simulink model "A_Robot_2_0_m_5_V22_SI"  (R2025b)
settings: Solver=VariableStepAuto  StartTime=0.0  StopTime=150  RelTol=1e-3
model workspace (MAT data in the model file):
  Km = [1; 1]
values from neighbouring files (symbols this model uses):
  kcl = kil + 50    (= 75)    [A_init_0.m]    (also in A_init_0_v2.m; A_init_1_v2.m)
  kcr = kir + 50    (= 75)    [A_init_0.m]    (also in A_init_0_v2.m; A_init_1_v2.m)
  kil = 25    [A_init_0.m]    (also in A_init_0_v2.m; A_init_1_v2.m)
  kir = 25    [A_init_0.m]    (also in A_init_0_v2.m; A_init_1_v2.m)
  kpl = 5    [A_init_0.m]    (also in A_init_0_v2.m; A_init_1_v2.m)
  kpr = 5    [A_init_0.m]    (also in A_init_0_v2.m; A_init_1_v2.m)
  theta0 = theta_0_min + (theta_0_max - theta_0_min) * rand()    [A_init_0.m]    (also in A_init_0_v2.m; A_init_1_v2.m)
  theta_gsr = theta_gsr_min + (theta_gsr_max - theta_gsr_min) * rand()    [A_init_0.m]    (also in A_init_0_v2.m; A_init_1_v2.m)
  v_rand = v_rand_0 + (v_rand_max - v_rand_0) * rand()    [A_init_0.m]    (also in A_init_0_v2.m; A_init_1_v2.m)
  x0 = x_0_min + (x_0_max - x_0_min) * rand()    [A_init_0.m]    (also in A_init_0_v2.m; A_init_1_v2.m)
  x_gsr = x_gsr_min + (x_gsr_max - x_gsr_min) * rand()    [A_init_0.m]    (also in A_init_0_v2.m; A_init_1_v2.m)
  y0 = y_0_min + (y_0_max - y_0_min) * rand()    [A_init_0.m]    (also in A_init_0_v2.m; A_init_1_v2.m)
  y_gsr = y_gsr_min + (y_gsr_max - y_gsr_min) * rand()    [A_init_0.m]    (also in A_init_0_v2.m; A_init_1_v2.m)
undefined symbols (not defined in the file or in its folder): DiscIntNeverNeededParam
libraries: simulink x15, rllib x1
(part 1 of 3)
settings Model: PacingRate=10  Creator=rafci  LastModifiedBy=rafci
settings DataIOCC: InspectSignalLogs=on
settings DebuggingCC: AlgebraicLoopMsg=none

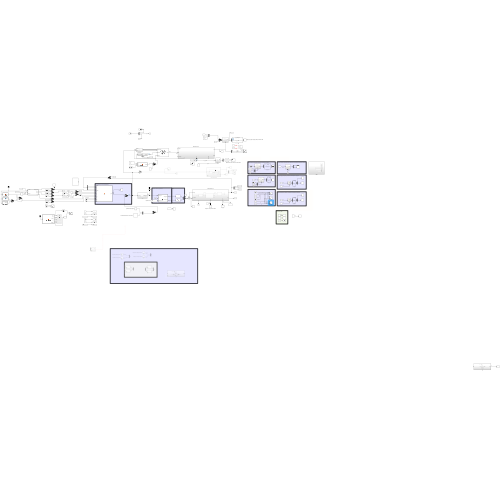
[thumbnail: Simulink's stored preview of the top-level diagram]
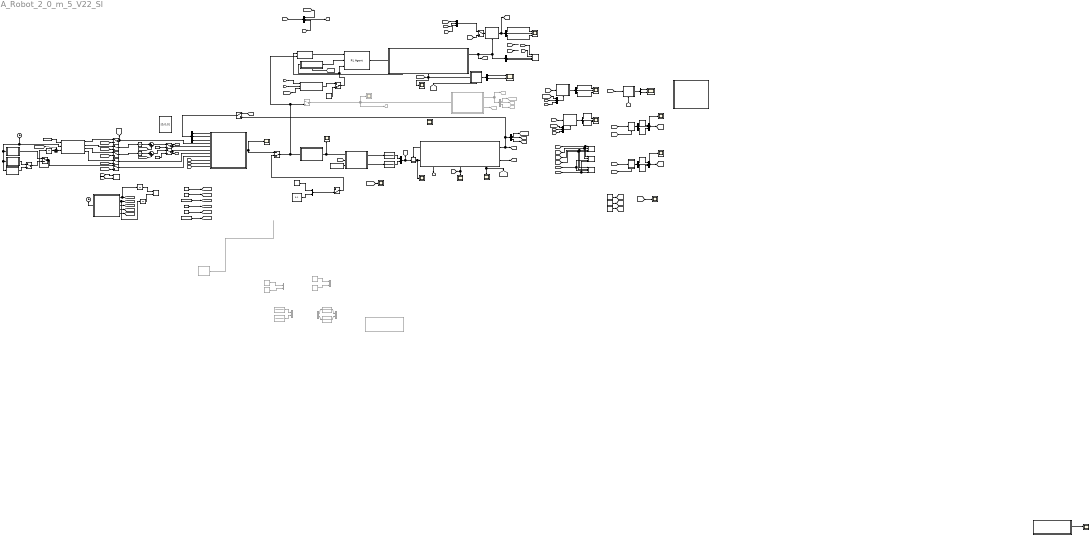
== system A_Robot_2_0_m_5_V22_SI ==
  note: Wykresy XY
  note: Błąd pozycji pomiędzy modelem kinematyki a GSR
  note: Błąd pozycji pomiędzy modelem kinematyki a pełnym
  note: Roznica napięć pomiędzy sterowaniem kinematyki a pełnego modelu
  note: $\Omega_{dsF}$
  note: FIltry
  note: parametry ASP
  note: Kinematyczny steownik platformy
  note: Blok sterowania prędkości
  note: Błąd prędkości pomiędzy modelem kinematyki a pełnym
  note: Błąd pozycji pomiędzy pełnym modelem a GSR
  Błąd napięć między pełnym modelem a NN : Scope  NumInputPorts=2
      settings: ActiveDisplayYMinimum=-28.46005  ActiveDisplayYMaximum=16.49556
  Błąd pozycji i kąta między (switch) modelem a NN : Scope  NumInputPorts=3
      settings: ActiveDisplayYMinimum=-0.50596  ActiveDisplayYMaximum=0.10747
  Clock : Clock
  Clock1 : Clock
  Constant : Constant  Value=10  VectorParams1D=off
  Constant1 : Constant  Value=40
  Constant10 : Constant  Value=x_gsr
  Constant11 : Constant  Value=y_gsr
  Constant12 : Constant  Value=theta_gsr
  Constant13 : Constant  Value=[0;0;0]
  Constant2 : Constant  Value=27
  Constant3 : Constant  Value=x0
  Constant4 : Constant  Value=y0
  Constant5 : Constant  Value=0  OutDataTypeStr=boolean
  Constant6 : Constant  Value=theta0
  Constant7 : Constant  Value=-0.5
  Constant8 : Constant  Value=-0.5
  Constant9 : Constant  Value=v_rand
  Demux : Demux  Commented=on  Outputs=3
  Demux{1..3,5,7..9,11..12} (9 alike) : Demux  Outputs=3
  Demux13 : Demux  Outputs=2
  Demux4 : Demux  Commented=on  Outputs=2
  Demux6 : Demux  Outputs=2
  Goto11 : Goto  Commented=on  GotoTag=U_k  TagVisibility=global
  Goto12 : Goto  Commented=on  GotoTag=q_k  TagVisibility=global
  Goto16 : Goto  Commented=on  GotoTag=q_d_k  TagVisibility=global
  Goto17 : Goto  Commented=on  GotoTag=theta_k  TagVisibility=global
  Goto18 : Goto  Commented=on  GotoTag=x_k  TagVisibility=global
  Goto19 : Goto  Commented=on  GotoTag=y_k  TagVisibility=global
  Integrator{,1,6..8} (5 alike) : Integrator
  J^-1 : Subsystem
  MATLAB Function : MATLAB Function  TreatAsAtomicUnit=on
  MATLAB Function1 : MATLAB Function  TreatAsAtomicUnit=on
  MATLAB Function10 : MATLAB Function  TreatAsAtomicUnit=on
  MATLAB Function2 : MATLAB Function  TreatAsAtomicUnit=on
  MATLAB Function3 : MATLAB Function  TreatAsAtomicUnit=on
  MATLAB Function6 : MATLAB Function  TreatAsAtomicUnit=on
  MATLAB Function7 : MATLAB Function  TreatAsAtomicUnit=on
  MATLAB Function9 : MATLAB Function  TreatAsAtomicUnit=on
  Manual Switch{,2..3,5..10,12,15} (11 alike) : ManualSwitch
  Manual Switch11 : ManualSwitch  CurrentSetting=0
  Manual Switch13 : ManualSwitch  Commented=on
  Manual Switch14 : ManualSwitch  CurrentSetting=0
  Manual Switch4 : ManualSwitch  CurrentSetting=0
  Model Robota 2.0 : Subsystem
      settings: PortSchema="{\"entries\":[{\"content\":{\"sides\":[{\"content\":{\"connectorIds\":[\"Out6\",\"In1\"]},\"type\":\"ConnectorPlacement.EquallySpacedRectSide\",\"uuid\":\"c09d05f6-15bd-4af9-8cdd-7798699522a1\"},{\"content\":{\"connectorIds\":[\"Out1\",\"Out2\"],\"side\":\"RIGHT\"},\"type\":\"ConnectorPlacement.EquallySpacedRectSide\",\"uuid\":\"5078d491-052a-42da-8be8-27dff9332d53\"},{\"content\":{\"side\":\"TOP\"},\"type\":\"ConnectorPlacement.EquallySpacedRectSide\",\"uuid\":\"ce1dd30c-527c-4a1c-9b39-bff6482988ba\"},{\"content\":{\"connectorIds\":[\"Out3\",\"Out4\",\"Out5\"],\"side\":\"BOTTOM\"},\"type\":\"ConnectorPlacement.EquallySpacedRectSide\",\"uuid\":\"43230f6c-2d05-4ed1-a059-067bd37565f0\"}]},\"type\":\"ConnectorPlacement.EquallySpacedConnector\",\"uuid\":\"daca06f7-ab0b-4c67-a969-f3b079c7dee2\"}],\"packageUris\":[\"http://schema.mathworks.com/mf0/Connector/R2020b\"],\"version\":\"1.0\"}"
  Model Robota 2.1 : Subsystem
      settings: PortSchema="{\"entries\":[{\"content\":{\"sides\":[{\"content\":{\"connectorIds\":[\"Out6\",\"In1\",\"In2\"]},\"type\":\"ConnectorPlacement.EquallySpacedRectSide\",\"uuid\":\"c09d05f6-15bd-4af9-8cdd-7798699522a1\"},{\"content\":{\"connectorIds\":[\"Out1\",\"Out2\"],\"side\":\"RIGHT\"},\"type\":\"ConnectorPlacement.EquallySpacedRectSide\",\"uuid\":\"5078d491-052a-42da-8be8-27dff9332d53\"},{\"content\":{\"side\":\"TOP\"},\"type\":\"ConnectorPlacement.EquallySpacedRectSide\",\"uuid\":\"ce1dd30c-527c-4a1c-9b39-bff6482988ba\"},{\"content\":{\"connectorIds\":[\"Out3\",\"Out4\",\"Out5\"],\"side\":\"BOTTOM\"},\"type\":\"ConnectorPlacement.EquallySpacedRectSide\",\"uuid\":\"43230f6c-2d05-4ed1-a059-067bd37565f0\"}]},\"type\":\"ConnectorPlacement.EquallySpacedConnector\",\"uuid\":\"daca06f7-ab0b-4c67-a969-f3b079c7dee2\"}],\"packageUris\":[\"http://schema.mathworks.com/mf0/Connector/R2020b\"],\"version\":\"1.0\"}"
  Model kinematyki1 : Subsystem  Commented=on
  Mux1 : Mux  Inputs=2
  Mux{3,6,8,10} (4 alike) : Mux  Commented=on  Inputs=2
  Mux{4..5,7,9,12} (5 alike) : Mux  Inputs=3
  Mux2 : Mux  Inputs=2
  Nagroda : Subsystem
      settings: PortSchema="{\"entries\":[{\"content\":{\"sides\":[{\"content\":{\"connectorIds\":[\"In1\"]},\"type\":\"ConnectorPlacement.EquallySpacedRectSide\",\"uuid\":\"a2f775dc-59c4-4717-86d2-15fa652a3e96\"},{\"content\":{\"connectorIds\":[\"Out1\"],\"side\":\"RIGHT\"},\"type\":\"ConnectorPlacement.EquallySpacedRectSide\",\"uuid\":\"245f7467-b166-487e-99c9-5f03cfbee592\"},{\"content\":{\"side\":\"TOP\"},\"type\":\"ConnectorPlacement.EquallySpacedRectSide\",\"uuid\":\"946a6bdb-83a2-4b9a-b4f9-a3cb3678f859\"},{\"content\":{\"connectorIds\":[\"In2\"],\"side\":\"BOTTOM\"},\"type\":\"ConnectorPlacement.EquallySpacedRectSide\",\"uuid\":\"f1f94bb1-6799-4829-990b-56c54b864c73\"}]},\"type\":\"ConnectorPlacement.EquallySpacedConnector\",\"uuid\":\"54b4897f-7a99-44dc-b2f7-11c656f05ccb\"}],\"packageUris\":[\"http://schema.mathworks.com/mf0/Connector/R2020b\"],\"version\":\"1.0\"}"
  Napięcie na lewym silniku : Constant  Commented=on  Value=12
  "Napięcie na prawym silniku " : Constant  Commented=on  Value=70
  Napięcie na wejsciowe silników : Scope
      settings: ActiveDisplayYMinimum=-5.36622  ActiveDisplayYMaximum=6.84937  DataLoggingVariableName=ScopeData8
  Obsrwacja : Subsystem
  Prędkość Lewego wału : Constant  Commented=on  Value=0
  Prędkość max : Constant  Value=161.77*2*pi
  Prędkość prawego wału : Constant  Commented=on  Value=75
  RL Agent : rllib/RL Agent  Agent=agent  ExternalActionAsInput=off  ProvideLastAction=off  ProvideCumRwd=off  TreatAsDirectFeedthrough=on  UseStrictObservationDataTypes=off
  Scope{,1..3,5..6,8,11,17,20} (10 alike) : Scope
      Scope1 settings: ActiveDisplayYMinimum=-0.01608  ActiveDisplayYMaximum=0.01608  DataLoggingVariableName=ScopeData7
      Scope11 settings: ActiveDisplayYMinimum=-0.23934  ActiveDisplayYMaximum=0.23817  DataLoggingVariableName=ScopeData7
      Scope17 settings: ActiveDisplayYMinimum=-2.83473  ActiveDisplayYMaximum=3.59922
      Scope2 settings: ActiveDisplayYMinimum=-0.01608  ActiveDisplayYMaximum=0.01608  DataLoggingVariableName=ScopeData10
      Scope20 settings: ActiveDisplayYMinimum=-0.01395  ActiveDisplayYMaximum=0.11266  DataLoggingVariableName=ScopeData2
      Scope3 settings: ActiveDisplayYMinimum=-0.0233  ActiveDisplayYMaximum=0.04203
      Scope5 settings: ActiveDisplayYMinimum=-6.16909  ActiveDisplayYMaximum=6.96286  DataLoggingVariableName=ScopeData2
      Scope6 settings: ActiveDisplayYMinimum=2.8655866160988808  ActiveDisplayYMaximum=3.93364068120718
      Scope8 settings: ActiveDisplayYMinimum=-0.02162  ActiveDisplayYMaximum=0.2946
      Scope settings: ActiveDisplayYMinimum=-0.48296536475593865  ActiveDisplayYMaximum=4.3057020124132714
  Scope12 : Scope  Commented=on
      settings: ActiveDisplayYMinimum=-0.0125  ActiveDisplayYMaximum=0.1125  DataLoggingVariableName=ScopeData8
  Scope24 : Scope  NumInputPorts=3
      settings: ActiveDisplayYMinimum=-0.06798  ActiveDisplayYMaximum=0.06446  DataLoggingVariableName=ScopeData5
  Scope4 : Scope  NumInputPorts=3
      settings: ActiveDisplayYMinimum=-0.1993  ActiveDisplayYMaximum=0.19665
  Scope9 : Scope  NumInputPorts=2
      settings: ActiveDisplayYMinimum=-0.4921  ActiveDisplayYMaximum=2.2769  DataLoggingVariableName=ScopeData6
  Stałe : Subsystem
  Subsystem : Subsystem  Commented=on
  Subsystem1 : Subsystem  Commented=on
      settings: PortSchema="{\"entries\":[{\"content\":{\"sides\":[{\"content\":{\"connectorIds\":[\"In1\"]},\"type\":\"ConnectorPlacement.EquallySpacedRectSide\",\"uuid\":\"f81facd5-8dce-4a5d-a044-cb75bd1df10e\"},{\"content\":{\"connectorIds\":[\"Out1\"],\"side\":\"RIGHT\"},\"type\":\"ConnectorPlacement.EquallySpacedRectSide\",\"uuid\":\"361c4912-9b0e-4ff4-a4c3-0f951cd83b7e\"},{\"content\":{\"side\":\"TOP\"},\"type\":\"ConnectorPlacement.EquallySpacedRectSide\",\"uuid\":\"7c64f9f2-ca51-41c2-8f6b-bbae03c31185\"},{\"content\":{\"connectorIds\":[\"In2\"],\"side\":\"BOTTOM\"},\"type\":\"ConnectorPlacement.EquallySpacedRectSide\",\"uuid\":\"00962904-9a33-4c86-93c6-1e958d83cf78\"}]},\"type\":\"ConnectorPlacement.EquallySpacedConnector\",\"uuid\":\"b3c5fd64-8318-4fc9-b064-dcb9a80ffa17\"}],\"packageUris\":[\"http://schema.mathworks.com/mf0/Connector/R2020b\"],\"version\":\"1.0\"}"
  Subsystem10 : Subsystem
      settings: PortSchema="{\"entries\":[{\"content\":{\"sides\":[{\"content\":{\"connectorIds\":[\"In1\"]},\"type\":\"ConnectorPlacement.EquallySpacedRectSide\",\"uuid\":\"f81facd5-8dce-4a5d-a044-cb75bd1df10e\"},{\"content\":{\"connectorIds\":[\"Out1\"],\"side\":\"RIGHT\"},\"type\":\"ConnectorPlacement.EquallySpacedRectSide\",\"uuid\":\"361c4912-9b0e-4ff4-a4c3-0f951cd83b7e\"},{\"content\":{\"side\":\"TOP\"},\"type\":\"ConnectorPlacement.EquallySpacedRectSide\",\"uuid\":\"7c64f9f2-ca51-41c2-8f6b-bbae03c31185\"},{\"content\":{\"connectorIds\":[\"In2\"],\"side\":\"BOTTOM\"},\"type\":\"ConnectorPlacement.EquallySpacedRectSide\",\"uuid\":\"00962904-9a33-4c86-93c6-1e958d83cf78\"}]},\"type\":\"ConnectorPlacement.EquallySpacedConnector\",\"uuid\":\"b3c5fd64-8318-4fc9-b064-dcb9a80ffa17\"}],\"packageUris\":[\"http://schema.mathworks.com/mf0/Connector/R2020b\"],\"version\":\"1.0\"}"
  Subsystem2 : Subsystem
      settings: PortSchema="{\"entries\":[{\"content\":{\"sides\":[{\"content\":{\"connectorIds\":[\"In1\"]},\"type\":\"ConnectorPlacement.EquallySpacedRectSide\",\"uuid\":\"f81facd5-8dce-4a5d-a044-cb75bd1df10e\"},{\"content\":{\"connectorIds\":[\"Out1\"],\"side\":\"RIGHT\"},\"type\":\"ConnectorPlacement.EquallySpacedRectSide\",\"uuid\":\"361c4912-9b0e-4ff4-a4c3-0f951cd83b7e\"},{\"content\":{\"connectorIds\":[\"In2\"],\"side\":\"TOP\"},\"type\":\"ConnectorPlacement.EquallySpacedRectSide\",\"uuid\":\"7c64f9f2-ca51-41c2-8f6b-bbae03c31185\"}]},\"type\":\"ConnectorPlacement.EquallySpacedConnector\",\"uuid\":\"b3c5fd64-8318-4fc9-b064-dcb9a80ffa17\"}],\"packageUris\":[\"http://schema.mathworks.com/mf0/Connector/R2020b\"],\"version\":\"1.0\"}"
  Subsystem3 : Subsystem
      settings: PortSchema="{\"entries\":[{\"content\":{\"sides\":[{\"content\":{\"connectorIds\":[\"In1\"]},\"type\":\"ConnectorPlacement.EquallySpacedRectSide\",\"uuid\":\"f81facd5-8dce-4a5d-a044-cb75bd1df10e\"},{\"content\":{\"connectorIds\":[\"Out1\"],\"side\":\"RIGHT\"},\"type\":\"ConnectorPlacement.EquallySpacedRectSide\",\"uuid\":\"361c4912-9b0e-4ff4-a4c3-0f951cd83b7e\"},{\"content\":{\"side\":\"TOP\"},\"type\":\"ConnectorPlacement.EquallySpacedRectSide\",\"uuid\":\"7c64f9f2-ca51-41c2-8f6b-bbae03c31185\"},{\"content\":{\"connectorIds\":[\"In2\"],\"side\":\"BOTTOM\"},\"type\":\"ConnectorPlacement.EquallySpacedRectSide\",\"uuid\":\"00962904-9a33-4c86-93c6-1e958d83cf78\"}]},\"type\":\"ConnectorPlacement.EquallySpacedConnector\",\"uuid\":\"b3c5fd64-8318-4fc9-b064-dcb9a80ffa17\"}],\"packageUris\":[\"http://schema.mathworks.com/mf0/Connector/R2020b\"],\"version\":\"1.0\"}"
  Subsystem4 : Subsystem
      settings: PortSchema="{\"entries\":[{\"content\":{\"sides\":[{\"content\":{\"connectorIds\":[\"In1\"]},\"type\":\"ConnectorPlacement.EquallySpacedRectSide\",\"uuid\":\"f81facd5-8dce-4a5d-a044-cb75bd1df10e\"},{\"content\":{\"connectorIds\":[\"Out1\"],\"side\":\"RIGHT\"},\"type\":\"ConnectorPlacement.EquallySpacedRectSide\",\"uuid\":\"361c4912-9b0e-4ff4-a4c3-0f951cd83b7e\"},{\"content\":{\"side\":\"TOP\"},\"type\":\"ConnectorPlacement.EquallySpacedRectSide\",\"uuid\":\"7c64f9f2-ca51-41c2-8f6b-bbae03c31185\"},{\"content\":{\"connectorIds\":[\"In2\"],\"side\":\"BOTTOM\"},\"type\":\"ConnectorPlacement.EquallySpacedRectSide\",\"uuid\":\"00962904-9a33-4c86-93c6-1e958d83cf78\"}]},\"type\":\"ConnectorPlacement.EquallySpacedConnector\",\"uuid\":\"b3c5fd64-8318-4fc9-b064-dcb9a80ffa17\"}],\"packageUris\":[\"http://schema.mathworks.com/mf0/Connector/R2020b\"],\"version\":\"1.0\"}"
  Subsystem5 : Subsystem
      settings: PortSchema="{\"entries\":[{\"content\":{\"sides\":[{\"content\":{\"connectorIds\":[\"In1\"]},\"type\":\"ConnectorPlacement.EquallySpacedRectSide\",\"uuid\":\"f81facd5-8dce-4a5d-a044-cb75bd1df10e\"},{\"content\":{\"connectorIds\":[\"Out1\"],\"side\":\"RIGHT\"},\"type\":\"ConnectorPlacement.EquallySpacedRectSide\",\"uuid\":\"361c4912-9b0e-4ff4-a4c3-0f951cd83b7e\"},{\"content\":{\"side\":\"TOP\"},\"type\":\"ConnectorPlacement.EquallySpacedRectSide\",\"uuid\":\"7c64f9f2-ca51-41c2-8f6b-bbae03c31185\"},{\"content\":{\"connectorIds\":[\"In2\"],\"side\":\"BOTTOM\"},\"type\":\"ConnectorPlacement.EquallySpacedRectSide\",\"uuid\":\"00962904-9a33-4c86-93c6-1e958d83cf78\"}]},\"type\":\"ConnectorPlacement.EquallySpacedConnector\",\"uuid\":\"b3c5fd64-8318-4fc9-b064-dcb9a80ffa17\"}],\"packageUris\":[\"http://schema.mathworks.com/mf0/Connector/R2020b\"],\"version\":\"1.0\"}"
  Subsystem6 : Subsystem
      settings: PortSchema="{\"entries\":[{\"content\":{\"sides\":[{\"content\":{\"connectorIds\":[\"In1\"]},\"type\":\"ConnectorPlacement.EquallySpacedRectSide\",\"uuid\":\"f81facd5-8dce-4a5d-a044-cb75bd1df10e\"},{\"content\":{\"connectorIds\":[\"Out1\"],\"side\":\"RIGHT\"},\"type\":\"ConnectorPlacement.EquallySpacedRectSide\",\"uuid\":\"361c4912-9b0e-4ff4-a4c3-0f951cd83b7e\"},{\"content\":{\"side\":\"TOP\"},\"type\":\"ConnectorPlacement.EquallySpacedRectSide\",\"uuid\":\"7c64f9f2-ca51-41c2-8f6b-bbae03c31185\"},{\"content\":{\"connectorIds\":[\"In2\"],\"side\":\"BOTTOM\"},\"type\":\"ConnectorPlacement.EquallySpacedRectSide\",\"uuid\":\"00962904-9a33-4c86-93c6-1e958d83cf78\"}]},\"type\":\"ConnectorPlacement.EquallySpacedConnector\",\"uuid\":\"b3c5fd64-8318-4fc9-b064-dcb9a80ffa17\"}],\"packageUris\":[\"http://schema.mathworks.com/mf0/Connector/R2020b\"],\"version\":\"1.0\"}"
  Subsystem7 : Subsystem
      settings: PortSchema="{\"entries\":[{\"content\":{\"sides\":[{\"content\":{\"connectorIds\":[\"In1\"]},\"type\":\"ConnectorPlacement.EquallySpacedRectSide\",\"uuid\":\"f81facd5-8dce-4a5d-a044-cb75bd1df10e\"},{\"content\":{\"connectorIds\":[\"Out1\"],\"side\":\"RIGHT\"},\"type\":\"ConnectorPlacement.EquallySpacedRectSide\",\"uuid\":\"361c4912-9b0e-4ff4-a4c3-0f951cd83b7e\"},{\"content\":{\"side\":\"TOP\"},\"type\":\"ConnectorPlacement.EquallySpacedRectSide\",\"uuid\":\"7c64f9f2-ca51-41c2-8f6b-bbae03c31185\"},{\"content\":{\"connectorIds\":[\"In2\"],\"side\":\"BOTTOM\"},\"type\":\"ConnectorPlacement.EquallySpacedRectSide\",\"uuid\":\"00962904-9a33-4c86-93c6-1e958d83cf78\"}]},\"type\":\"ConnectorPlacement.EquallySpacedConnector\",\"uuid\":\"b3c5fd64-8318-4fc9-b064-dcb9a80ffa17\"}],\"packageUris\":[\"http://schema.mathworks.com/mf0/Connector/R2020b\"],\"version\":\"1.0\"}"
  Subsystem8 : Subsystem
      settings: PortSchema="{\"entries\":[{\"content\":{\"sides\":[{\"content\":{\"connectorIds\":[\"In1\"]},\"type\":\"ConnectorPlacement.EquallySpacedRectSide\",\"uuid\":\"f81facd5-8dce-4a5d-a044-cb75bd1df10e\"},{\"content\":{\"connectorIds\":[\"Out1\"],\"side\":\"RIGHT\"},\"type\":\"ConnectorPlacement.EquallySpacedRectSide\",\"uuid\":\"361c4912-9b0e-4ff4-a4c3-0f951cd83b7e\"},{\"content\":{\"side\":\"TOP\"},\"type\":\"ConnectorPlacement.EquallySpacedRectSide\",\"uuid\":\"7c64f9f2-ca51-41c2-8f6b-bbae03c31185\"},{\"content\":{\"connectorIds\":[\"In2\"],\"side\":\"BOTTOM\"},\"type\":\"ConnectorPlacement.EquallySpacedRectSide\",\"uuid\":\"00962904-9a33-4c86-93c6-1e958d83cf78\"}]},\"type\":\"ConnectorPlacement.EquallySpacedConnector\",\"uuid\":\"b3c5fd64-8318-4fc9-b064-dcb9a80ffa17\"}],\"packageUris\":[\"http://schema.mathworks.com/mf0/Connector/R2020b\"],\"version\":\"1.0\"}"
  Subsystem9 : Subsystem
      settings: PortSchema="{\"entries\":[{\"content\":{\"sides\":[{\"content\":{\"connectorIds\":[\"In1\"]},\"type\":\"ConnectorPlacement.EquallySpacedRectSide\",\"uuid\":\"f81facd5-8dce-4a5d-a044-cb75bd1df10e\"},{\"content\":{\"connectorIds\":[\"Out1\"],\"side\":\"RIGHT\"},\"type\":\"ConnectorPlacement.EquallySpacedRectSide\",\"uuid\":\"361c4912-9b0e-4ff4-a4c3-0f951cd83b7e\"},{\"content\":{\"side\":\"TOP\"},\"type\":\"ConnectorPlacement.EquallySpacedRectSide\",\"uuid\":\"7c64f9f2-ca51-41c2-8f6b-bbae03c31185\"},{\"content\":{\"connectorIds\":[\"In2\"],\"side\":\"BOTTOM\"},\"type\":\"ConnectorPlacement.EquallySpacedRectSide\",\"uuid\":\"00962904-9a33-4c86-93c6-1e958d83cf78\"}]},\"type\":\"ConnectorPlacement.EquallySpacedConnector\",\"uuid\":\"b3c5fd64-8318-4fc9-b064-dcb9a80ffa17\"}],\"packageUris\":[\"http://schema.mathworks.com/mf0/Connector/R2020b\"],\"version\":\"1.0\"}"
  Sum : Sum  Inputs=|++
  Sum1 : Sum  Inputs=|++
  Sum2 : Sum  Inputs=++|
  Transfer Fcn : TransferFcn  Commented=on  Numerator=[9.4]  Denominator=[0.094 1]
  Transfer Fcn1 : TransferFcn  Denominator=[0.016 1]
  Transfer Fcn2 : TransferFcn  Denominator=[0.016 1]
  Transfer Fcn3 : TransferFcn  Commented=on  Numerator=[9.4]  Denominator=[0.094 1]
  Transfer Fcn4 : TransferFcn  Commented=on  Denominator=[0.016 1]
  Transfer Fcn5 : TransferFcn  Commented=on  Denominator=[0.016 1]
  U_m_e : Scope
      settings: ActiveDisplayYMinimum=-0.61452  ActiveDisplayYMaximum=0.7843  DataLoggingVariableName=ScopeData9
  XY Graph : Record  NumPorts=4.0  FileSettingsInternal="{\"entries\":[{\"content\":{\"excelSettings\":{\"content\":{},\"type\":\"Streamout.ExcelSettings\"},\"parquetSettings\":{\"content\":{},\"type\":\"Streamout.ParquetSettings\"}},\"type\":\"Streamout.FileSettingStorage\",\"uuid\":\"\"}],\"packageUris\":[\"http:\\/\\/schema.mathworks.com\\/mf0\\/streamout_blocks\\/R2020a\"],\"version\":\"1.0\"}"  FrameSettings=[0, 0, 0, 0]  Layout=[1 1]  SignalsInternal="{\"entries\":[{\"content\":{\"signals\":[{\"content\":{\"blockPath\":[],\"dimensions\":[1],\"domain\":\"\",\"lineColor\":\"#77ac30\",\"lineWidth\":2,\"plots\":[ 1 ],\"port\":3,\"sid\":[\"\"],\"signalID\":1,\"signalName\":\"x\"},\"type\":\"RecordBlkView.Signal\",\"uuid\":\"\"},{\"content\":{\"blockPath\":[],\"dimensions\":[1],\"domain\":\"\",\"lineColor\":\"#4dbeee\",\"lineWidth\":2,\"plots\":[ 1 ],\"port\":4,\"sid\":[\"\"],\"signalID\":2,\"signalName\":\"y\"},\"type\":\"RecordBlkView.Signal\",\"uuid\":\"\"},{\"content\":{\"blockPath\":[],\"dimensions\":[1],\"domain\":\"\",\"lineColor\":\"#edb120\",\"lineWidth\":2,\"plots\":[ 1 ],\"port\":1,\"sid\":[\"\"],\"signalID\":3,\"signalName\":\"x_k\"},\"type\":\"RecordBlkView.Signal\",\"uuid\":\"\"},{\"content\":{\"blockPath\":[],\"dimensions\":[1],\"domain\":\"\",\"lineColor\":\"#7e2f8e\",\"lineWidth\":2,\"plots\":[ 1 ],\"port\":2,\"sid\":[\"\"],\"signalID\":4,\"signalName\":\"y_k\"},\"type\":\"RecordBlkView.Signal\",\"uuid\":\"\"}]},\"type\":\"RecordBlkView.InputSignals\",\"uuid\":\"\"}],\"packageUris\":[\"http:\\/\\/schema.mathworks.com\\/mf0\\/streamout_blocks\\/R2020a\"],\"version\":\"1.0\"}"  VisualizationBindings="{\"xyplotplugin\":{\"info\":[{\"series\":[{\"bindingParametersList\":[{\"parameter\":\"X-Axis\",\"signalID\":3,\"signalName\":\"x_k\"},{\"parameter\":\"Y-Axis\",\"signalID\":4,\"signalName\":\"y_k\"}],\"seriesID\":0},{\"bindingParametersList\":[{\"parameter\":\"X-Axis\",\"signalID\":1,\"signalName\":\"x\"},{\"parameter\":\"Y-Axis\",\"signalID\":2,\"signalName\":\"y\"}],\"seriesID\":1}],\"subplotID\":1}]}}"  CompatibilityTag=XY
  XY Graph1 : Record  NumPorts=2.0  FileSettingsInternal="{\"entries\":[{\"content\":{\"excelSettings\":{\"content\":{},\"type\":\"Streamout.ExcelSettings\"},\"parquetSettings\":{\"content\":{},\"type\":\"Streamout.ParquetSettings\"}},\"type\":\"Streamout.FileSettingStorage\",\"uuid\":\"\"}],\"packageUris\":[\"http:\\/\\/schema.mathworks.com\\/mf0\\/streamout_blocks\\/R2020a\"],\"version\":\"1.0\"}"  FrameSettings=[0, 0]  Layout=[1 1]  SignalsInternal="{\"entries\":[{\"content\":{\"signals\":[{\"content\":{\"blockPath\":[],\"dimensions\":[1],\"domain\":\"\",\"lineColor\":\"#fe330a\",\"lineWidth\":2,\"plots\":[ 1 ],\"port\":1,\"sid\":[\"\"],\"signalID\":1,\"signalName\":\"From33\"},\"type\":\"RecordBlkView.Signal\",\"uuid\":\"\"},{\"content\":{\"blockPath\":[],\"dimensions\":[1],\"domain\":\"\",\"lineColor\":\"#22b573\",\"lineWidth\":2,\"plots\":[ 1 ],\"port\":2,\"sid\":[\"\"],\"signalID\":2,\"signalName\":\"From34\"},\"type\":\"RecordBlkView.Signal\",\"uuid\":\"\"}]},\"type\":\"RecordBlkView.InputSignals\",\"uuid\":\"\"}],\"packageUris\":[\"http:\\/\\/schema.mathworks.com\\/mf0\\/streamout_blocks\\/R2020a\"],\"version\":\"1.0\"}"  VisualizationBindings="{\"xyplotplugin\":{\"info\":[{\"series\":[{\"bindingParametersList\":[{\"parameter\":\"X-Axis\",\"signalID\":1,\"signalName\":\"From33\"},{\"parameter\":\"Y-Axis\",\"signalID\":2,\"signalName\":\"From34\"}],\"seriesID\":0}],\"subplotID\":1}]}}"  CompatibilityTag=XY
  XY Graph2 : Record  NumPorts=4.0  FileSettingsInternal="{\"entries\":[{\"content\":{\"excelSettings\":{\"content\":{},\"type\":\"Streamout.ExcelSettings\"},\"parquetSettings\":{\"content\":{},\"type\":\"Streamout.ParquetSettings\"}},\"type\":\"Streamout.FileSettingStorage\",\"uuid\":\"\"}],\"packageUris\":[\"http:\\/\\/schema.mathworks.com\\/mf0\\/streamout_blocks\\/R2020a\"],\"version\":\"1.0\"}"  FrameSettings=[0, 0, 0, 0]  Layout=[1 1]  SignalsInternal="{\"entries\":[{\"content\":{\"signals\":[{\"content\":{\"blockPath\":[],\"dimensions\":[1],\"domain\":\"\",\"lineColor\":\"#edb120\",\"lineWidth\":2,\"port\":3,\"sid\":[\"\"],\"signalID\":1,\"signalName\":\"xr\"},\"type\":\"RecordBlkView.Signal\",\"uuid\":\"\"},{\"content\":{\"blockPath\":[],\"dimensions\":[1],\"domain\":\"\",\"lineColor\":\"#7e2f8e\",\"lineWidth\":2,\"port\":4,\"sid\":[\"\"],\"signalID\":2,\"signalName\":\"yr\"},\"type\":\"RecordBlkView.Signal\",\"uuid\":\"\"},{\"content\":{\"blockPath\":[],\"dimensions\":[1],\"domain\":\"\",\"lineColor\":\"#edb120\",\"lineWidth\":2,\"port\":1,\"sid\":[\"\"],\"signalID\":3,\"signalName\":\"x_k\"},\"type\":\"RecordBlkView.Signal\",\"uuid\":\"\"},{\"content\":{\"blockPath\":[],\"dimensions\":[1],\"domain\":\"\",\"lineColor\":\"#7e2f8e\",\"lineWidth\":2,\"port\":2,\"sid\":[\"\"],\"signalID\":4,\"signalName\":\"y_k\"},\"type\":\"RecordBlkView.Signal\",\"uuid\":\"\"}]},\"type\":\"RecordBlkView.InputSignals\",\"uuid\":\"\"}],\"packageUris\":[\"http:\\/\\/schema.mathworks.com\\/mf0\\/streamout_blocks\\/R2020a\"],\"version\":\"1.0\"}"  VisualizationBindings="{\"xyplotplugin\":{\"info\":[{\"series\":[],\"subplotID\":1}]}}"  CompatibilityTag=XY
  XY Graph3 : Record  NumPorts=4.0  FileSettingsInternal="{\"entries\":[{\"content\":{\"excelSettings\":{\"content\":{},\"type\":\"Streamout.ExcelSettings\"},\"parquetSettings\":{\"content\":{},\"type\":\"Streamout.ParquetSettings\"}},\"type\":\"Streamout.FileSettingStorage\",\"uuid\":\"\"}],\"packageUris\":[\"http:\\/\\/schema.mathworks.com\\/mf0\\/streamout_blocks\\/R2020a\"],\"version\":\"1.0\"}"  FrameSettings=[0, 0, 0, 0]  Layout=[1 1]  SignalsInternal="{\"entries\":[{\"content\":{\"signals\":[{\"content\":{\"blockPath\":[],\"dimensions\":[1],\"domain\":\"\",\"lineColor\":\"#22b573\",\"lineWidth\":2,\"plots\":[ 1 ],\"port\":1,\"sid\":[\"\"],\"signalID\":1,\"signalName\":\"x\"},\"type\":\"RecordBlkView.Signal\",\"uuid\":\"\"},{\"content\":{\"blockPath\":[],\"dimensions\":[1],\"domain\":\"\",\"lineColor\":\"#22b573\",\"lineWidth\":2,\"plots\":[ 1 ],\"port\":2,\"sid\":[\"\"],\"signalID\":2,\"signalName\":\"y\"},\"type\":\"RecordBlkView.Signal\",\"uuid\":\"\"},{\"content\":{\"blockPath\":[],\"dimensions\":[1],\"domain\":\"\",\"lineColor\":\"#a2142f\",\"lineWidth\":2,\"plots\":[ 1 ],\"port\":3,\"sid\":[\"\"],\"signalID\":3,\"signalName\":\"xr\"},\"type\":\"RecordBlkView.Signal\",\"uuid\":\"\"},{\"content\":{\"blockPath\":[],\"dimensions\":[1],\"domain\":\"\",\"lineColor\":\"#d95319\",\"lineWidth\":2,\"plots\":[ 1 ],\"port\":4,\"sid\":[\"\"],\"signalID\":4,\"signalName\":\"yr\"},\"type\":\"RecordBlkView.Signal\",\"uuid\":\"\"}]},\"type\":\"RecordBlkView.InputSignals\",\"uuid\":\"\"}],\"packageUris\":[\"http:\\/\\/schema.mathworks.com\\/mf0\\/streamout_blocks\\/R2020a\"],\"version\":\"1.0\"}"  VisualizationBindings="{\"xyplotplugin\":{\"info\":[{\"series\":[{\"bindingParametersList\":[{\"parameter\":\"X-Axis\",\"signalID\":1,\"signalName\":\"x\"},{\"parameter\":\"Y-Axis\",\"signalID\":2,\"signalName\":\"y\"}],\"seriesID\":0},{\"bindingParametersList\":[{\"parameter\":\"X-Axis\",\"signalID\":3,\"signalName\":\"xr\"},{\"parameter\":\"Y-Axis\",\"signalID\":4,\"signalName\":\"yr\"}],\"seriesID\":1}],\"subplotID\":1}]}}"  CompatibilityTag=XY
  XY Graph4 : Record  NumPorts=2.0  FileSettingsInternal="{\"entries\":[{\"content\":{\"excelSettings\":{\"content\":{},\"type\":\"Streamout.ExcelSettings\"},\"parquetSettings\":{\"content\":{},\"type\":\"Streamout.ParquetSettings\"}},\"type\":\"Streamout.FileSettingStorage\",\"uuid\":\"\"}],\"packageUris\":[\"http:\\/\\/schema.mathworks.com\\/mf0\\/streamout_blocks\\/R2020a\"],\"version\":\"1.0\"}"  FrameSettings=[0, 0]  Layout=[1 1]  SignalsInternal="{\"entries\":[{\"content\":{\"signals\":[{\"content\":{\"blockPath\":[],\"dimensions\":[1],\"domain\":\"\",\"lineColor\":\"#ff6929\",\"lineWidth\":2,\"port\":1,\"sid\":[\"\"],\"signalID\":1,\"signalName\":\"Integrator\"},\"type\":\"RecordBlkView.Signal\",\"uuid\":\"\"},{\"content\":{\"blockPath\":[],\"dimensions\":[1],\"domain\":\"\",\"lineColor\":\"#b746ff\",\"lineWidth\":2,\"port\":2,\"sid\":[\"\"],\"signalID\":2,\"signalName\":\"Integrator1\"},\"type\":\"RecordBlkView.Signal\",\"uuid\":\"\"}]},\"type\":\"RecordBlkView.InputSignals\",\"uuid\":\"\"}],\"packageUris\":[\"http:\\/\\/schema.mathworks.com\\/mf0\\/streamout_blocks\\/R2020a\"],\"version\":\"1.0\"}"  VisualizationBindings="{\"xyplotplugin\":{\"info\":[{\"series\":[],\"subplotID\":1}]}}"  CompatibilityTag=XY
  XY PI a NN : Record  NumPorts=4.0  FileSettingsInternal="{\"entries\":[{\"content\":{\"excelSettings\":{\"content\":{},\"type\":\"Streamout.ExcelSettings\"},\"parquetSettings\":{\"content\":{},\"type\":\"Streamout.ParquetSettings\"}},\"type\":\"Streamout.FileSettingStorage\",\"uuid\":\"\"}],\"packageUris\":[\"http:\\/\\/schema.mathworks.com\\/mf0\\/streamout_blocks\\/R2020a\"],\"version\":\"1.0\"}"  FrameSettings=[0, 0, 0, 0]  Layout=[1 1]  SignalsInternal="{\"entries\":[{\"content\":{\"signals\":[{\"content\":{\"blockPath\":[],\"dimensions\":[1],\"domain\":\"\",\"lineColor\":\"#22b573\",\"lineWidth\":2,\"plots\":[ 1 ],\"port\":1,\"sid\":[\"\"],\"signalID\":1,\"signalName\":\"xr\"},\"type\":\"RecordBlkView.Signal\",\"uuid\":\"\"},{\"content\":{\"blockPath\":[],\"dimensions\":[1],\"domain\":\"\",\"lineColor\":\"#22b573\",\"lineWidth\":2,\"plots\":[ 1 ],\"port\":2,\"sid\":[\"\"],\"signalID\":2,\"signalName\":\"xy\"},\"type\":\"RecordBlkView.Signal\",\"uuid\":\"\"},{\"content\":{\"blockPath\":[],\"dimensions\":[1],\"domain\":\"\",\"lineColor\":\"#ff13a6\",\"lineWidth\":2,\"plots\":[ 1 ],\"port\":3,\"sid\":[\"\"],\"signalID\":3,\"signalName\":\"x_NN\"},\"type\":\"RecordBlkView.Signal\",\"uuid\":\"\"},{\"content\":{\"blockPath\":[],\"dimensions\":[1],\"domain\":\"\",\"lineColor\":\"#ff13a6\",\"lineWidth\":2,\"plots\":[ 1 ],\"port\":4,\"sid\":[\"\"],\"signalID\":4,\"signalName\":\"y_NN\"},\"type\":\"RecordBlkView.Signal\",\"uuid\":\"\"}]},\"type\":\"RecordBlkView.InputSignals\",\"uuid\":\"\"}],\"packageUris\":[\"http:\\/\\/schema.mathworks.com\\/mf0\\/streamout_blocks\\/R2020a\"],\"version\":\"1.0\"}"  VisualizationBindings="{\"xyplotplugin\":{\"info\":[{\"series\":[{\"bindingParametersList\":[{\"parameter\":\"X-Axis\",\"signalID\":3,\"signalName\":\"x_NN\"},{\"parameter\":\"Y-Axis\",\"signalID\":4,\"signalName\":\"y_NN\"}],\"seriesID\":0},{\"bindingParametersList\":[{\"parameter\":\"X-Axis\",\"signalID\":1,\"signalName\":\"xr\"},{\"parameter\":\"Y-Axis\",\"signalID\":2,\"signalName\":\"xy\"}],\"seriesID\":1}],\"subplotID\":1}]}}"  CompatibilityTag=XY
  prędkość kątowa [rad/s] : Constant  Value=0
  prędkość liniowa [m/s] (max=0.0151) : Constant  Value=0.1
  tag scope: E_NN=global, U=global, U_m=global, U_m_NN=global, U_m_e=global, dxo=global, dyo=global, e_theta=global, e_x=global, e_y=global, k1=global, k2=global, k3=global, omegado=global, q=global, q_NN=global, q_d=global, theta0=global, theta=global, theta_gsr=global, thetao=global, thetar=global, vdo=global, x0=global, x=global, x_gsr=global, xr=global, y0=global, y=global, y_gsr=global, yr=global
  wires:
  prędkość kątowa [rad/s]/1 -> Mux1/1
  prędkość liniowa [m/s] (max=0.0151)/1 -> Mux1/2
  Napięcie na lewym silniku/1 -> Mux3/2  "U_mL"
  "Napięcie na prawym silniku "/1 -> Mux3/1  "U_mR"
  Prędkość max/1 -> MATLAB Function6/3(omega_m_max)
  [ng] -> MATLAB Function6/2(ng)
  Clock/1 -> MATLAB Function10/1(t), MATLAB Function1/1(t), MATLAB Function2/1(t), MATLAB Function9/2(t)
  Prędkość prawego wału/1 -> Mux8/1  "wdc_R"
  Prędkość Lewego wału/1 -> Mux8/2  "wdc_L"
  Demux3/3 -> MATLAB Function7/3(y)
  Integrator6/1 -> Sum2/2
  MATLAB Function6/2(omega_dsL) -> Transfer Fcn2/1  "wds_L"
  Transfer Fcn4/1 -> Mux10/1
  Transfer Fcn5/1 -> Mux10/2
  Constant/1 -> [k1]
  Constant1/1 -> [k2]
  Constant2/1 -> [k3]
  [k1] -> MATLAB Function7/9(k1)
  [k3] -> MATLAB Function7/11(k3)
  [k2] -> MATLAB Function7/10(k2)
  MATLAB Function7/1(u_dc) -> Manual Switch4/1, Scope8/1
  MATLAB Function6/1(omega_dsP) -> Transfer Fcn1/1  "wds_R"
  Demux4/2 -> Transfer Fcn3/1
  Demux4/1 -> Transfer Fcn/1
  Transfer Fcn/1 -> Mux6/1
  Transfer Fcn3/1 -> Mux6/2
  Manual Switch2/1 -> MATLAB Function7/5(xr), [xr]
  Manual Switch3/1 -> MATLAB Function7/6(yr), [yr]
  Integrator7/1 -> Sum/1
  Constant3/1 -> [x0]
  Constant4/1 -> [y0]
  Integrator8/1 -> Sum1/1
  Demux3/2 -> MATLAB Function7/2(x)
  Subsystem2/1(Out) -> Scope11/1, Model Robota 2.0/1(E_omega)
  Model Robota 2.0/6(Omega) -> Subsystem2/2(-)
  Transfer Fcn2/1 -> Mux2/2
  Transfer Fcn1/1 -> Mux2/1
  Model kinematyki1/1(q) -> Demux/1, Goto12/1
  Manual Switch15/1 -> Demux3/1
  [e_q] -> Scope3/1
  Mux2/1 -> Subsystem2/1(+), [omegadsF]  "OmegadsF"
  [omegadsF] -> Scope5/1
  Subsystem5/1(Out) -> Demux6/1
  Manual Switch4/1 -> J^-1/1(u_dc), Manual Switch13/2, Obsrwacja/2(U_dc)
  [x_k] -> XY Graph2/1, XY Graph/1  "x_k"
  [yr] -> XY Graph2/4, XY Graph3/4  "yr"
  [xr] -> XY Graph2/3, XY Graph3/3  "xr"
  Subsystem8/1(Out) -> Demux9/1
  Demux9/1 -> Scope24/1  "e_r_theta_k"
  Demux8/2 -> Mux12/2  "e_x"
  Demux9/2 -> Scope24/2  "e_r_x_k"
  [thetar] -> Mux7/1
  Mux7/1 -> Subsystem8/2(-1)
  Demux8/1 -> Mux12/1  "e_theta"
  [xr] -> Mux7/2
  Demux8/3 -> Mux12/3  "e_y"
  [y_k] -> XY Graph2/2, XY Graph/2  "y_k"
  Demux9/3 -> Scope24/3  "e_r_y_k"
  Subsystem9/1(Out) -> Scope20/1
  [yr] -> Mux7/3
  Model Robota 2.0/3(u) -> [U]
  Model Robota 2.0/4(U_m) -> Napięcie na wejsciowe silników/1, [U_m]  "U_m"
  Model Robota 2.0/5(U_me) -> U_m_e/1, [U_m_e]
  [U_k] -> Subsystem5/1(+)  "U_m_k"
  [U] -> Subsystem5/2(-)  "U_m"
  Subsystem7/1(Out) -> Demux8/1
  Mux12/1 -> Scope1/1, [e_q]
  [q_k] -> Subsystem7/1(+)
  [q] -> Subsystem7/2(-)
  [q_d] -> Subsystem3/2(-)
  [q_d_k] -> Subsystem3/1(+)
  Mux4/1 -> Scope2/1, [e_q_d]
  Subsystem3/1(Out) -> Demux1/1
  Demux1/2 -> Mux4/2  "e_xd"
  Demux1/3 -> Mux4/3  "e_yd"
  Demux1/1 -> Mux4/1  "e_thetad"
  Model Robota 2.0/2(dq) -> [q_d]
  Model kinematyki1/2(dq) -> Goto16/1
  Subsystem4/1(Out) -> Demux2/1
  Demux2/1 -> Scope4/1  "e_r_theta"
  [xr] -> Mux5/2
  [thetar] -> Mux5/1
  Demux2/3 -> Scope4/3  "e_r_y"
  [yr] -> Mux5/3
  Mux5/1 -> Subsystem4/2(-1)
  Demux2/2 -> Scope4/2  "e_r_x"
  [q_k] -> Subsystem8/1(+)
  [q] -> Subsystem4/1(+)
  Demux/1 -> Goto17/1
  Demux/2 -> Goto18/1
  Demux/3 -> Goto19/1
  Demux5/1 -> [theta]
  Demux5/2 -> [x]
  Demux5/3 -> [y]
  [y] -> XY Graph3/2, XY Graph/4  "y"
  [x] -> XY Graph3/1, XY Graph/3  "x"
  J^-1/1(Omega_dc) -> MATLAB Function6/1(omega_dc), Scope17/1
  Demux3/1 -> MATLAB Function7/1(theta)
  Subsystem/1(u_dc) -> ?
  Clock1/1 -> MATLAB Function/1(t)
  MATLAB Function/3(theta_r) -> [thetao]
  Manual Switch5/1 -> Integrator7/1
  Manual Switch6/1 -> Integrator8/1
  Manual Switch7/1 -> MATLAB Function7/7(vr)
  [thetao] -> Manual Switch/2
  [dxo] -> Manual Switch5/2
  [dyo] -> Manual Switch6/2
  [vdo] -> Manual Switch7/2
  MATLAB Function9/1(theta_d_out) -> Manual Switch/1
  MATLAB Function9/2(dx_d) -> Manual Switch5/1
  MATLAB Function9/3(dy_d) -> Manual Switch6/1
  MATLAB Function9/4(v_d) -> Manual Switch7/1
  MATLAB Function/5(omega_r) -> [omegado]
  [omegado] -> Manual Switch8/2
  Manual Switch8/1 -> MATLAB Function7/8(wr)
  MATLAB Function/2(dy_r) -> Integrator1/1, [dyo]
  MATLAB Function/4(v_r) -> [vdo]
  MATLAB Function/1(dx_r) -> Integrator/1, [dxo]
  MATLAB Function10/1(dtheta_d) -> Manual Switch9/1
  MATLAB Function1/1(dtheta_d) -> Manual Switch10/1
  Manual Switch9/1 -> Manual Switch8/1, Integrator6/1
  [yr] -> XY Graph1/2
  [xr] -> XY Graph1/1
  MATLAB Function2/1(dtheta_d) -> Manual Switch10/2
  Manual Switch10/1 -> Manual Switch9/2
  Integrator/1 -> XY Graph4/1
  Integrator1/1 -> XY Graph4/2
  Demux6/1 -> Scope9/1  "E_m_r"
  Demux6/2 -> Scope9/2  "E_m_l"
  Mux1/1 -> Manual Switch11/2
  Manual Switch11/1 -> Manual Switch4/2
  Demux7/1 -> [e_theta]  "e_theta"
  Demux7/2 -> [e_x]  "e_x"
  [q] -> Manual Switch12/2
  Demux11/3 -> Błąd pozycji i kąta między (switch) modelem a NN/3  "e_r_y_NN"
  Subsystem6/1(Out) -> [E_NN], Demux11/1
  Demux11/2 -> Błąd pozycji i kąta między (switch) modelem a NN/2  "e_r_x_NN"
  Demux11/1 -> Błąd pozycji i kąta między (switch) modelem a NN/1  "e_r_theta_NN"
  Model Robota 2.1/1(q) -> [q_NN], Demux12/1, Subsystem6/2(-1)
  [x] -> ?  "x"
  [y] -> ?  "y"
  Demux12/3 -> XY PI a NN/4  "y_NN"
  Demux12/2 -> XY PI a NN/3  "x_NN"
  Subsystem10/1(Out) -> Demux13/1
  [U_m] -> Subsystem10/2(-)  "U_m"
  Demux13/2 -> Błąd napięć między pełnym modelem a NN/2  "E_m_l_NN"
  Demux13/1 -> Błąd napięć między pełnym modelem a NN/1  "E_m_r_NN"
  Model Robota 2.1/4(U_m) -> Scope6/1, [U_m_NN], Subsystem10/1(+)  "U_m_NN"
  Manual Switch12/1 -> Subsystem6/1(+)
  Mux9/1 -> Manual Switch12/1
  Demux7/3 -> [e_y]  "e_y"
  Nagroda/1(reward) -> RL Agent/2  "nagroda"
  [e_theta] -> MATLAB Function3/3(e_theta)
  [e_x] -> MATLAB Function3/1(e_x)
  [e_y] -> MATLAB Function3/2(e_y)
  RL Agent/1 -> Model Robota 2.1/1(NN)
  [yr] -> Mux9/3
  [xr] -> Mux9/2
  [thetar] -> Mux9/1
  Model Robota 2.1/3(u) -> Obsrwacja/1(U_NN)
  Obsrwacja/1(Out1) -> RL Agent/1
  Manual Switch13/1 -> Goto11/1, Model kinematyki1/1(u), Scope12/1
  [E_NN] -> Demux7/1
  [U_m_NN] -> Nagroda/2(U)
  Manual Switch14/1 -> RL Agent/3, Nagroda/1(spad z rowerka)
  MATLAB Function3/1(done) -> Manual Switch14/1
  Constant5/1 -> Manual Switch14/2
  Model Robota 2.0/1(q) -> Manual Switch15/2, Demux5/1, [q]
  [q_NN] -> Manual Switch15/1
  [yr] -> XY PI a NN/2  "xy"
  [xr] -> XY PI a NN/1  "xr"
  Sum1/1 -> Manual Switch3/1
  Sum/1 -> Manual Switch2/1
  [y_gsr] -> Sum1/2
  [x_gsr] -> Sum/2
  Constant6/1 -> [theta0]
  [theta_gsr] -> Sum2/1
  Manual Switch/1 -> [thetar], MATLAB Function7/4(thetar)
  Constant7/1 -> Manual Switch2/2
  Constant8/1 -> Manual Switch3/2
  Sum2/1 -> MATLAB Function9/3(theta_d)
  Constant9/1 -> MATLAB Function9/1(v_rand)
  Constant12/1 -> [theta_gsr]
  Constant10/1 -> [x_gsr]
  Constant11/1 -> [y_gsr]

== system A_Robot_2_0_m_5_V22_SI/J^-1 ==
  u_dc : Inport
  MATLAB Function8 : MATLAB Function  TreatAsAtomicUnit=on
  Omega_dc : Outport
  wires:
  [b] -> MATLAB Function8/3(b)
  [r] -> MATLAB Function8/2(r)
  u_dc/1 -> MATLAB Function8/1(u_dc)
  MATLAB Function8/1(Omega_dc) -> Omega_dc/1

== system A_Robot_2_0_m_5_V22_SI/Model Robota 2.0 ==
  E_omega : Inport
  Model Dynamiki1 : Subsystem
  Model kinematyki1 : Subsystem
  regulator PI z korektorem anti-windup : Subsystem
  q : Outport
  dq : Outport  Port=2
  u : Outport  Port=3
  U_m : Outport  Port=4
  U_me : Outport  Port=5
  Omega : Outport  Port=6
  wires:
  E_omega/1 -> regulator PI z korektorem anti-windup/1(E_omega)
  Model kinematyki1/1(q) -> q/1
  Model Dynamiki1/1(u) -> Model kinematyki1/1(u), u/1
  Model kinematyki1/2(dq) -> dq/1
  Model Dynamiki1/2(Omega) -> Omega/1
  regulator PI z korektorem anti-windup/1(U_m) -> U_m/1, Model Dynamiki1/1(U_m)  "U_m"
  Model Dynamiki1/3(U_me) -> U_me/1

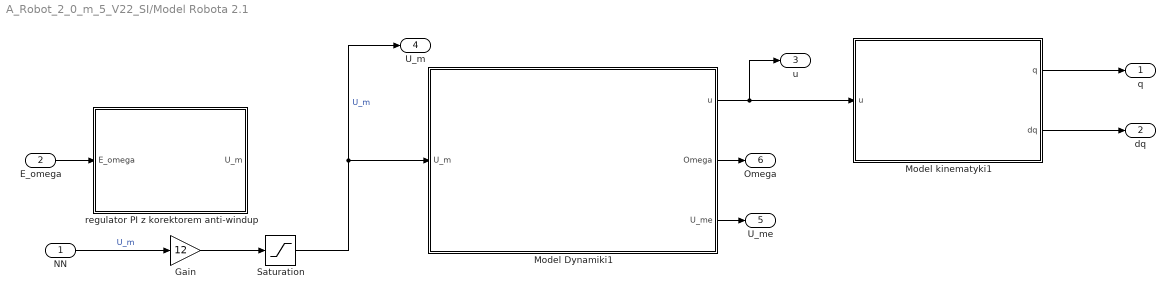
== system A_Robot_2_0_m_5_V22_SI/Model Robota 2.1 ==
  NN : Inport
  E_omega : Inport  Port=2
  Gain : Gain  Gain=12
  Model Dynamiki1 : Subsystem
  Model kinematyki1 : Subsystem
  Saturation : Saturate  UpperLimit=12  LowerLimit=-12
  regulator PI z korektorem anti-windup : Subsystem
  q : Outport
  dq : Outport  Port=2
  u : Outport  Port=3
  U_m : Outport  Port=4
  U_me : Outport  Port=5
  Omega : Outport  Port=6
  wires:
  E_omega/1 -> regulator PI z korektorem anti-windup/1(E_omega)
  Model kinematyki1/1(q) -> q/1
  Model Dynamiki1/1(u) -> u/1, Model kinematyki1/1(u)
  Model kinematyki1/2(dq) -> dq/1
  Model Dynamiki1/2(Omega) -> Omega/1
  Saturation/1 -> U_m/1, Model Dynamiki1/1(U_m)  "U_m"
  Model Dynamiki1/3(U_me) -> U_me/1
  NN/1 -> Gain/1  "U_m"
  Gain/1 -> Saturation/1

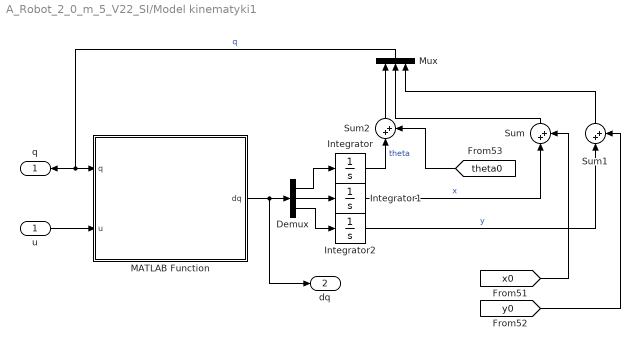
== system A_Robot_2_0_m_5_V22_SI/Model kinematyki1 ==
  u : Inport
  Demux : Demux  Outputs=3
  Integrator : Integrator
  Integrator1 : Integrator
  Integrator2 : Integrator
  MATLAB Function : MATLAB Function  TreatAsAtomicUnit=on
  Mux : Mux  Inputs=3
  Sum : Sum  Inputs=|++
  Sum1 : Sum  Inputs=|++
  Sum2 : Sum  Inputs=|++
  q : Outport
  dq : Outport  Port=2
  wires:
  Mux/1 -> q/1, MATLAB Function/1(q)  "q"
  Demux/1 -> Integrator/1
  Demux/3 -> Integrator2/1
  Demux/2 -> Integrator1/1
  Integrator2/1 -> Sum1/1  "y"
  MATLAB Function/1(dq) -> dq/1, Demux/1
  Integrator/1 -> Sum2/1  "theta"
  Integrator1/1 -> Sum/1  "x"
  u/1 -> MATLAB Function/2(u)
  [y0] -> Sum1/2
  [x0] -> Sum/2
  Sum/1 -> Mux/2
  Sum1/1 -> Mux/3
  [theta0] -> Sum2/2
  Sum2/1 -> Mux/1

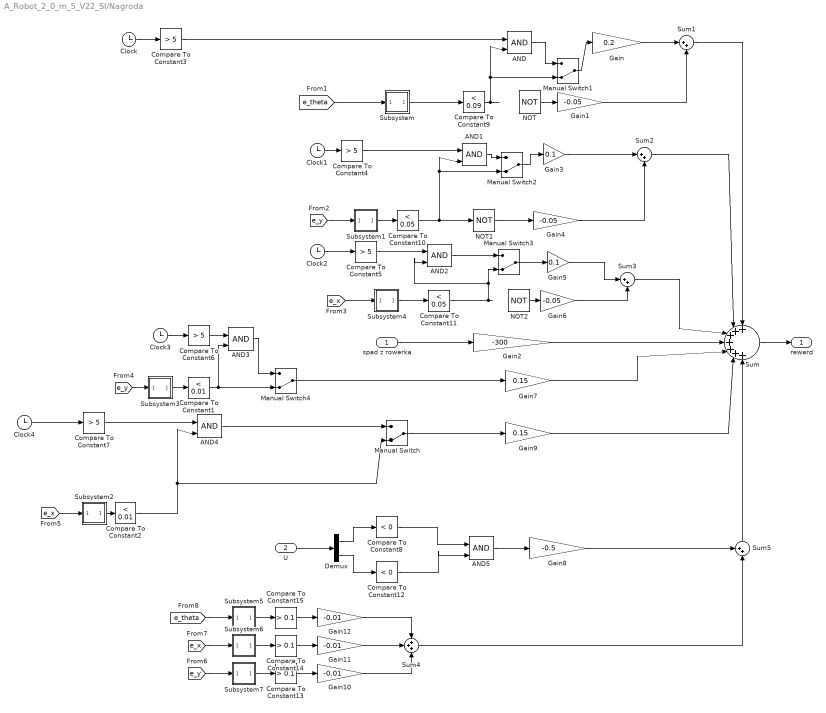
== system A_Robot_2_0_m_5_V22_SI/Nagroda ==
  spad z rowerka : Inport
  U : Inport  Port=2
  AND{,1..5} (6 alike) : Logic  IconShape=distinctive  AllPortsSameDT=off  OutDataTypeStr=boolean
  Clock{,1..4} (5 alike) : Clock
  Compare To Constant1 : simulink/Logic and Bit Operations/Compare To Constant  relop=<  const=0.01  OutDataTypeStr=boolean
  Compare To Constant10 : simulink/Logic and Bit Operations/Compare To Constant  relop=<  const=0.05  OutDataTypeStr=boolean
  Compare To Constant11 : simulink/Logic and Bit Operations/Compare To Constant  relop=<  const=0.05  OutDataTypeStr=boolean
  Compare To Constant12 : simulink/Logic and Bit Operations/Compare To Constant  relop=<  const=0  OutDataTypeStr=boolean
  Compare To Constant13 : simulink/Logic and Bit Operations/Compare To Constant  relop=>  const=0.1  OutDataTypeStr=boolean
  Compare To Constant14 : simulink/Logic and Bit Operations/Compare To Constant  relop=>  const=0.1  OutDataTypeStr=boolean
  Compare To Constant15 : simulink/Logic and Bit Operations/Compare To Constant  relop=>  const=0.1  OutDataTypeStr=boolean
  Compare To Constant2 : simulink/Logic and Bit Operations/Compare To Constant  relop=<  const=0.01  OutDataTypeStr=boolean
  Compare To Constant{3..7} (5 alike) : simulink/Logic and Bit Operations/Compare To Constant  relop=>  const=5  OutDataTypeStr=boolean
  Compare To Constant8 : simulink/Logic and Bit Operations/Compare To Constant  relop=<  const=0  OutDataTypeStr=boolean
  Compare To Constant9 : simulink/Logic and Bit Operations/Compare To Constant  relop=<  const=0.09  OutDataTypeStr=boolean
  Demux : Demux  Outputs=2
  Gain : Gain  Gain=0.2
  Gain1 : Gain  Gain=-0.05
  Gain10 : Gain  Gain=-0.01
  Gain11 : Gain  Gain=-0.01
  Gain12 : Gain  Gain=-0.01
  Gain2 : Gain  Gain=-300
  Gain3 : Gain  Gain=0.1
  Gain4 : Gain  Gain=-0.05
  Gain5 : Gain  Gain=0.1
  Gain6 : Gain  Gain=-0.05
  Gain7 : Gain  Gain=0.15
  Gain8 : Gain  Gain=-0.5
  Gain9 : Gain  Gain=0.15
  Manual Switch{,1..4} (5 alike) : ManualSwitch  CurrentSetting=0
  NOT : Logic  Operator=NOT  IconShape=distinctive  AllPortsSameDT=off  OutDataTypeStr=boolean
  NOT1 : Logic  Operator=NOT  IconShape=distinctive  AllPortsSameDT=off  OutDataTypeStr=boolean
  NOT2 : Logic  Operator=NOT  IconShape=distinctive  AllPortsSameDT=off  OutDataTypeStr=boolean
  Subsystem : Subsystem
  Subsystem1 : Subsystem
  Subsystem2 : Subsystem
  Subsystem3 : Subsystem
  Subsystem4 : Subsystem
  Subsystem5 : Subsystem
  Subsystem6 : Subsystem
  Subsystem7 : Subsystem
  Sum : Sum  Inputs=+++++++  OutDataTypeStr=double
  Sum1 : Sum  Inputs=|++
  Sum2 : Sum  Inputs=|++
  Sum3 : Sum  Inputs=|++
  Sum4 : Sum  Inputs=+++
  Sum5 : Sum  Inputs=++|
  reward : Outport  VectorParamsAs1DForOutWhenUnconnected=off
  wires:
  Manual Switch1/1 -> Gain/1
  NOT/1 -> Gain1/1
  Gain1/1 -> Sum1/2
  spad z rowerka/1 -> Gain2/1
  Sum/1 -> reward/1
  Gain2/1 -> Sum/4
  Compare To Constant9/1 -> AND/2, Manual Switch1/2
  [e_x] -> Subsystem4/1(In1)
  [e_y] -> Subsystem1/1(In1)
  Sum1/1 -> Sum/1
  Gain4/1 -> Sum2/2
  NOT1/1 -> Gain4/1
  Subsystem1/1(Out1) -> Compare To Constant10/1
  Gain3/1 -> Sum2/1
  Sum2/1 -> Sum/2
  Gain6/1 -> Sum3/2
  NOT2/1 -> Gain6/1
  Subsystem4/1(Out1) -> Compare To Constant11/1
  Gain5/1 -> Sum3/1
  Sum3/1 -> Sum/3
  [e_y] -> Subsystem3/1(In1)
  Subsystem3/1(Out1) -> Compare To Constant1/1
  Compare To Constant1/1 -> AND3/2, Manual Switch4/2
  Gain9/1 -> Sum/6
  Gain7/1 -> Sum/5
  [e_x] -> Subsystem2/1(In1)
  Compare To Constant2/1 -> AND4/2, Manual Switch/2
  AND/1 -> Manual Switch1/1
  Compare To Constant3/1 -> AND/1
  Clock/1 -> Compare To Constant3/1
  Compare To Constant4/1 -> AND1/1
  Clock1/1 -> Compare To Constant4/1
  Compare To Constant10/1 -> Manual Switch2/2, AND1/2, NOT1/1
  AND1/1 -> Manual Switch2/1
  Compare To Constant5/1 -> AND2/1
  Clock2/1 -> Compare To Constant5/1
  Compare To Constant11/1 -> Manual Switch3/2, AND2/2
  AND2/1 -> Manual Switch3/1
  Compare To Constant6/1 -> AND3/1
  Clock3/1 -> Compare To Constant6/1
  Manual Switch4/1 -> Gain7/1
  Compare To Constant7/1 -> AND4/1
  Clock4/1 -> Compare To Constant7/1
  Manual Switch/1 -> Gain9/1
  U/1 -> Demux/1
  Demux/1 -> Compare To Constant8/1
  Demux/2 -> Compare To Constant12/1
  Compare To Constant12/1 -> AND5/2
  Compare To Constant8/1 -> AND5/1
  AND5/1 -> Gain8/1
  AND4/1 -> Manual Switch/1
  Gain/1 -> Sum1/1
  Manual Switch2/1 -> Gain3/1
  Manual Switch3/1 -> Gain5/1
  AND3/1 -> Manual Switch4/1
  Subsystem7/1(Out1) -> Compare To Constant13/1
  [e_y] -> Subsystem7/1(In1)
  Compare To Constant13/1 -> Gain10/1
  [e_x] -> Subsystem6/1(In1)
  Subsystem6/1(Out1) -> Compare To Constant14/1
  Compare To Constant14/1 -> Gain11/1
  [e_theta] -> Subsystem5/1(In1)
  Subsystem5/1(Out1) -> Compare To Constant15/1
  Compare To Constant15/1 -> Gain12/1
  Gain11/1 -> Sum4/2
  Gain12/1 -> Sum4/1
  Gain10/1 -> Sum4/3
  Sum4/1 -> Sum5/2
  Gain8/1 -> Sum5/1
  Sum5/1 -> Sum/7
  [e_theta] -> Subsystem/1(In1)
  Subsystem/1(Out1) -> Compare To Constant9/1
  Subsystem2/1(Out1) -> Compare To Constant2/1

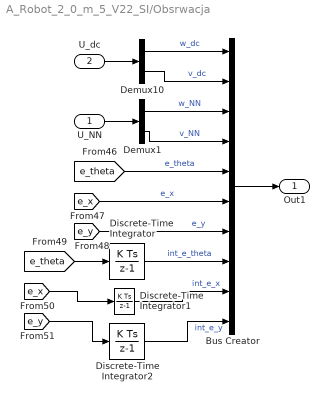
== system A_Robot_2_0_m_5_V22_SI/Obsrwacja ==
  U_NN : Inport
  U_dc : Inport  Port=2
  Bus Creator : BusCreator  Inputs=10
  Demux1 : Demux  Outputs=2
  Demux10 : Demux  Outputs=2
  Discrete-Time Integrator : DiscreteIntegrator  SampleTime=0.05  ICPrevOutput=DiscIntNeverNeededParam  ICPrevScaledInput=DiscIntNeverNeededParam
  Discrete-Time Integrator1 : DiscreteIntegrator  SampleTime=0.05  ICPrevOutput=DiscIntNeverNeededParam  ICPrevScaledInput=DiscIntNeverNeededParam
  Discrete-Time Integrator2 : DiscreteIntegrator  SampleTime=0.05  ICPrevOutput=DiscIntNeverNeededParam  ICPrevScaledInput=DiscIntNeverNeededParam
  Out1 : Outport
  wires:
  Demux1/2 -> Bus Creator/4  "v_NN"
  [e_theta] -> Discrete-Time Integrator/1
  [e_x] -> Discrete-Time Integrator1/1
  Discrete-Time Integrator1/1 -> Bus Creator/9  "int_e_x"
  Demux10/2 -> Bus Creator/2  "v_dc"
  Discrete-Time Integrator/1 -> Bus Creator/8  "int_e_theta"
  Discrete-Time Integrator2/1 -> Bus Creator/10  "int_e_y"
  Demux10/1 -> Bus Creator/1  "w_dc"
  Demux1/1 -> Bus Creator/3  "w_NN"
  [e_y] -> Discrete-Time Integrator2/1
  [e_x] -> Bus Creator/6  "e_x"
  [e_y] -> Bus Creator/7  "e_y"
  U_NN/1 -> Demux1/1
  Bus Creator/1 -> Out1/1
  U_dc/1 -> Demux10/1
  [e_theta] -> Bus Creator/5  "e_theta"

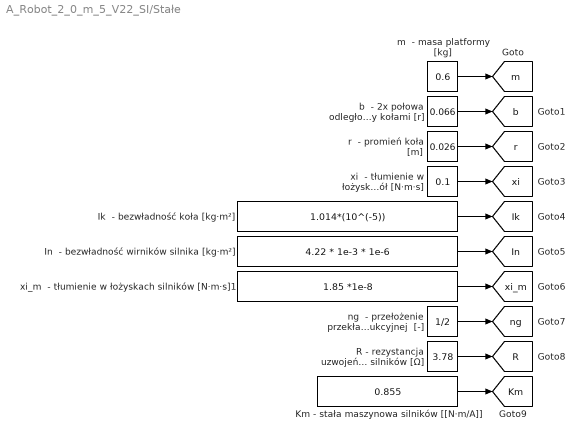
== system A_Robot_2_0_m_5_V22_SI/Stałe ==
  Ik  - bezwładność koła [kg·m²] : Constant  Value=1.014*(10^(-5))
  In  - bezwładność wirników silnika [kg·m²] : Constant  Value=4.22 * 1e-3 * 1e-6
  Km - stała maszynowa silników [[N·m/A]] : Constant  Value=0.855
  R - rezystancja uzwojeń silników [Ω] : Constant  Value=3.78
  b  - 2x połowa odległości między kołami [r] : Constant  Value=0.066
  m  - masa platformy [kg] : Constant  Value=0.6
  "ng  - przełożenie przekładni redukcyjnej  [-] " : Constant  Value=1/2
  r  - promień koła [m] : Constant  Value=0.026
  xi  - tłumienie w łożyskach kół [N·m·s] : Constant  Value=0.1
  xi_m  - tłumienie w łożyskach silników [N·m·s]1 : Constant  Value=1.85 *1e-8
  tag scope: Ik=global, In=global, Km=global, R=global, b=global, m=global, ng=global, r=global, xi=global, xi_m=global
  wires:
  xi_m  - tłumienie w łożyskach silników [N·m·s]1/1 -> [xi_m]
  R - rezystancja uzwojeń silników [Ω]/1 -> [R]
  "ng  - przełożenie przekładni redukcyjnej  [-] "/1 -> [ng]
  xi  - tłumienie w łożyskach kół [N·m·s]/1 -> [xi]
  Km - stała maszynowa silników [[N·m/A]]/1 -> [Km]
  b  - 2x połowa odległości między kołami [r]/1 -> [b]
  In  - bezwładność wirników silnika [kg·m²]/1 -> [In]
  m  - masa platformy [kg]/1 -> [m]
  r  - promień koła [m]/1 -> [r]
  Ik  - bezwładność koła [kg·m²]/1 -> [Ik]
